simulink model "pi_controller"  (R2022a)
settings: Solver=VariableStepAuto  StartTime=0.0  StopTime=30  RelTol=1e-3
libraries: simulink_extras x3
settings Model: Creator=pw705  LastModifiedBy=pw705

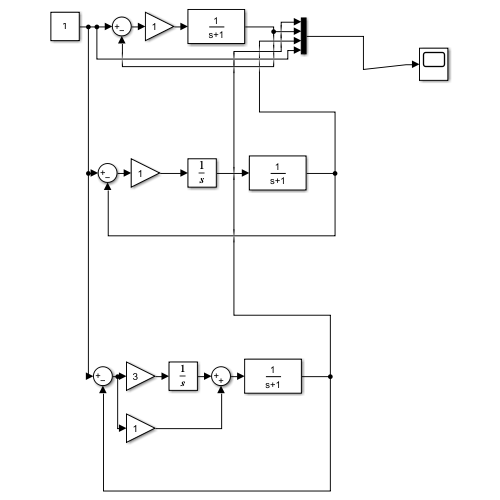
[thumbnail: Simulink's stored preview of the top-level diagram]
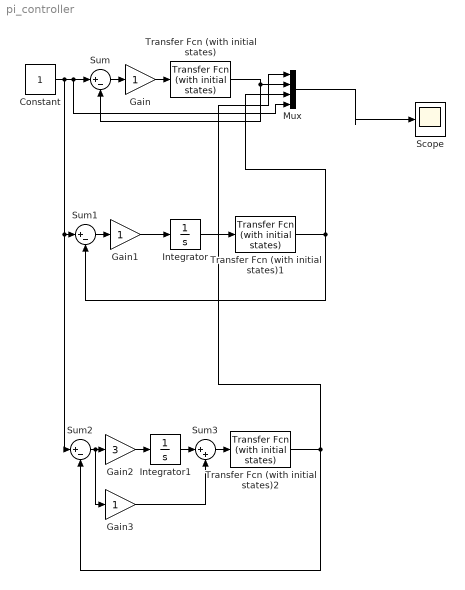
== system pi_controller ==
  Constant : Constant
  Gain : Gain
  Gain1 : Gain
  Gain2 : Gain  Gain=3
  Gain3 : Gain
  Integrator : Integrator
  Integrator1 : Integrator
  Mux : Mux
  Scope : Scope
  Sum : Sum  Inputs=|+-
  Sum1 : Sum  Inputs=|+-
  Sum2 : Sum  Inputs=|+-
  Sum3 : Sum  Inputs=|++
  Transfer Fcn (with initial states) : simulink_extras/Additional Linear/Transfer Fcn (with initial states)  N=[1]  D=[1 1]  X0=0
  Transfer Fcn (with initial states)1 : simulink_extras/Additional Linear/Transfer Fcn (with initial states)  N=[1]  D=[1 1]  X0=0
  Transfer Fcn (with initial states)2 : simulink_extras/Additional Linear/Transfer Fcn (with initial states)  N=[1]  D=[1 1]  X0=0
  wires:
  Sum/1 -> Gain/1
  Gain/1 -> Transfer Fcn (with initial states)/1
  Mux/1 -> Scope/1
  Transfer Fcn (with initial states)/1 -> Sum/2, Mux/2
  Gain1/1 -> Integrator/1
  Sum1/1 -> Gain1/1
  Constant/1 -> Sum2/1, Sum1/1, Mux/4, Sum/1
  Transfer Fcn (with initial states)1/1 -> Mux/3, Sum1/2
  Integrator/1 -> Transfer Fcn (with initial states)1/1
  Transfer Fcn (with initial states)2/1 -> Mux/1, Sum2/2
  Sum2/1 -> Gain3/1, Gain2/1
  Integrator1/1 -> Sum3/1
  Gain2/1 -> Integrator1/1
  Gain3/1 -> Sum3/2
  Sum3/1 -> Transfer Fcn (with initial states)2/1
